simulink model "FinalDJ"  (R2017a)
settings: Solver=VariableStepAuto  StartTime=0.0  StopTime=1000  RelTol=1e-3
undefined symbols (not defined in the file): fdesignblkfcn, gcbh
libraries: dspvision x4, dspsrcs4 x3, dspsigops x3, dspobslib x2
settings Model: Creator=ilyas  LastModifiedBy=ilyas

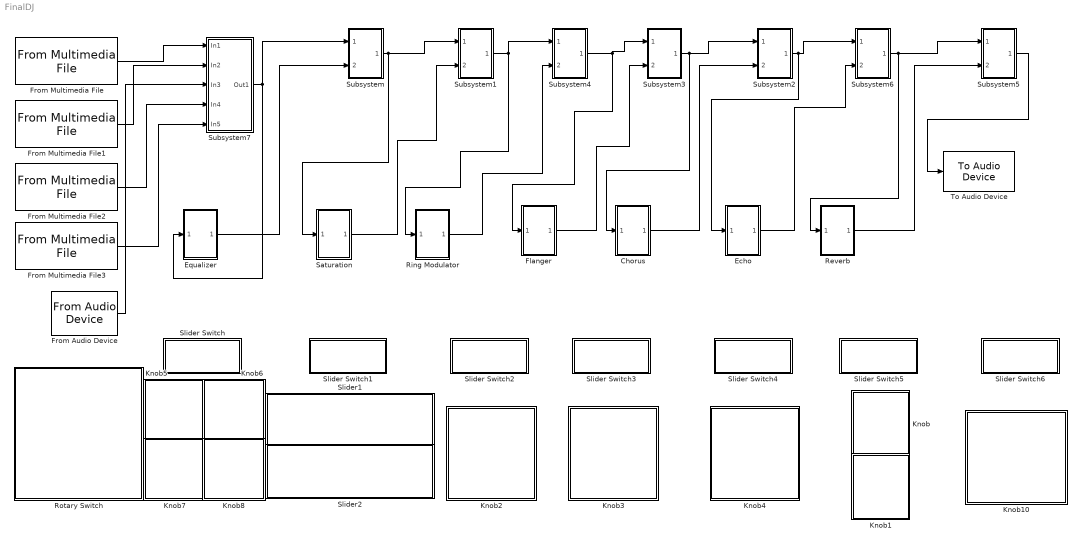
== system FinalDJ ==
  Chorus : Subsystem
  Echo : Subsystem
  Equalizer : Subsystem
  "Flanger " : Subsystem
  From Audio Device : dspobslib/From Audio Device  deviceName=Default  numChannels=1  sampleRate=44100  deviceDatatype=Determine from output data type  autoBufferSize=on  bufferSize=4096  queueDuration=1.0  frameSize=1024  outputDatatype=double  defaultInputChannelMapping=on  inputChannelMapping=1:2  outputNumOverrunSamples=off  OutputFrames=on
      settings: SourceProductName=DSP System Toolbox  SourceProductBaseCode=DS
  From Multimedia File : dspvision/From Multimedia File  inputFilename=C:\Users\ilyas\Desktop\cours UPMC\Son et image\audio\tpaudio\Tennessee-Whiskey-Cover-Instrumental-In-the-Style-.wav  loop=on  numPlays=inf  outputStreams=Audio only  videoDataType=single  audioDataType=double  inheritSampleTime=on  userDefinedSampleTime=1/30  noAudioOutput=off  isIntensityVideo=off  fourcc=RGB  colorVideoFormat=Separate color signals  outputEOF=off  dataOrg=Column-major  audioFrameSize=1024  computeAudioFrameSize=off  outSamplingMode=Sample based
      settings: SourceProductBaseCode=VP
  From Multimedia File1 : dspvision/From Multimedia File  inputFilename=C:\Users\ilyas\Desktop\cours UPMC\Son et image\audio\tpaudio\Comfortably_Numb_Pink_Floyd_Instrumental_Version_H.wav  loop=on  numPlays=inf  outputStreams=Audio only  videoDataType=single  audioDataType=double  inheritSampleTime=on  userDefinedSampleTime=1/30  noAudioOutput=off  isIntensityVideo=off  fourcc=RGB  colorVideoFormat=Separate color signals  outputEOF=off  dataOrg=Column-major  audioFrameSize=1024  computeAudioFrameSize=off  outSamplingMode=Sample based
      settings: SourceProductBaseCode=VP
  From Multimedia File2 : dspvision/From Multimedia File  inputFilename=C:\Users\ilyas\Desktop\cours UPMC\Son et image\audio\tpaudio\Perfect-Higher-Key-of-C-Piano-Karaoke-Instrumental.wav  loop=on  numPlays=inf  outputStreams=Audio only  videoDataType=single  audioDataType=double  inheritSampleTime=on  userDefinedSampleTime=1/30  noAudioOutput=off  isIntensityVideo=off  fourcc=RGB  colorVideoFormat=Separate color signals  outputEOF=off  dataOrg=Column-major  audioFrameSize=1024  computeAudioFrameSize=off  outSamplingMode=Sample based
      settings: SourceProductBaseCode=VP
  From Multimedia File3 : dspvision/From Multimedia File  inputFilename=C:\Users\ilyas\Desktop\cours UPMC\Son et image\audio\tpaudio\guitare.wav  loop=on  numPlays=inf  outputStreams=Audio only  videoDataType=single  audioDataType=double  inheritSampleTime=on  userDefinedSampleTime=1/30  noAudioOutput=off  isIntensityVideo=off  fourcc=RGB  colorVideoFormat=Separate color signals  outputEOF=off  dataOrg=Column-major  audioFrameSize=1024  computeAudioFrameSize=off  outSamplingMode=Sample based
      settings: SourceProductBaseCode=VP
  Knob : Subsystem  DialogController=hmiCreateDDGDialog  IsWebBlock=on  mask(MWDashboardBlock){webBlockId=d630c6b4-3853-4240-8efb-5ef3cca1801c, webBlockType=continuousknob, ShowInLibBrowser=on, ShowInitialText=on, HMISrcModelName=FinalDJ}
      mask prompts: webBlockId "WebBlock Id"; webBlockType "WebBlock Type"; HMISrcModelName "Source Model"
      mask help: SimulinkHMI:dialogs:ContinuousKnobDialogDesc
      mask Help: helpview([docroot '/mapfiles/simulink.map'], 'hmi_knob')
      mask Display:
      | if strcmp(get_param(bdroot(gcb),'BlockDiagramType'), 'library')
      |     image([(matlabroot) '/toolbox/simulink/hmi/icons/ContinuousKnob.png']);
      | end
  Knob1 : Subsystem  DialogController=hmiCreateDDGDialog  IsWebBlock=on  mask(MWDashboardBlock){webBlockId=0aec4347-f074-4d74-93b3-8d8c0f22ff46, webBlockType=continuousknob, ShowInLibBrowser=on, ShowInitialText=on, HMISrcModelName=FinalDJ}
      mask prompts: webBlockId "WebBlock Id"; webBlockType "WebBlock Type"; HMISrcModelName "Source Model"
      mask help: SimulinkHMI:dialogs:ContinuousKnobDialogDesc
      mask Help: helpview([docroot '/mapfiles/simulink.map'], 'hmi_knob')
      mask Display:
      | if strcmp(get_param(bdroot(gcb),'BlockDiagramType'), 'library')
      |     image([(matlabroot) '/toolbox/simulink/hmi/icons/ContinuousKnob.png']);
      | end
  Knob10 : Subsystem  DialogController=hmiCreateDDGDialog  IsWebBlock=on  mask(MWDashboardBlock){webBlockId=4e79f102-dad1-4d7d-9218-5af4294fe18a, webBlockType=continuousknob, ShowInLibBrowser=on, ShowInitialText=on, HMISrcModelName=FinalDJ}
      mask prompts: webBlockId "WebBlock Id"; webBlockType "WebBlock Type"; HMISrcModelName "Source Model"
      mask Help: helpview([docroot '/mapfiles/simulink.map'], 'hmi_knob')
      mask Display:
      | if strcmp(get_param(bdroot(gcb),'BlockDiagramType'), 'library')
      |     image([(matlabroot) '/toolbox/simulink/hmi/icons/ContinuousKnob.png']);
      | end
  Knob2 : Subsystem  DialogController=hmiCreateDDGDialog  IsWebBlock=on  mask(MWDashboardBlock){webBlockId=7d11c1b0-9d79-421c-bd63-6e862e6bd707, webBlockType=continuousknob, ShowInLibBrowser=on, ShowInitialText=on, HMISrcModelName=FinalDJ}
      mask prompts: webBlockId "WebBlock Id"; webBlockType "WebBlock Type"; HMISrcModelName "Source Model"
      mask help: SimulinkHMI:dialogs:ContinuousKnobDialogDesc
      mask Help: helpview([docroot '/mapfiles/simulink.map'], 'hmi_knob')
      mask Display:
      | if strcmp(get_param(bdroot(gcb),'BlockDiagramType'), 'library')
      |     image([(matlabroot) '/toolbox/simulink/hmi/icons/ContinuousKnob.png']);
      | end
  Knob3 : Subsystem  DialogController=hmiCreateDDGDialog  IsWebBlock=on  mask(MWDashboardBlock){webBlockId=41dfc1c3-3217-4a37-bd27-ffe62e9a6d62, webBlockType=continuousknob, ShowInLibBrowser=on, ShowInitialText=on, HMISrcModelName=FinalDJ}
      mask prompts: webBlockId "WebBlock Id"; webBlockType "WebBlock Type"; HMISrcModelName "Source Model"
      mask help: SimulinkHMI:dialogs:ContinuousKnobDialogDesc
      mask Help: helpview([docroot '/mapfiles/simulink.map'], 'hmi_knob')
      mask Display:
      | if strcmp(get_param(bdroot(gcb),'BlockDiagramType'), 'library')
      |     image([(matlabroot) '/toolbox/simulink/hmi/icons/ContinuousKnob.png']);
      | end
  Knob4 : Subsystem  DialogController=hmiCreateDDGDialog  IsWebBlock=on  mask(MWDashboardBlock){webBlockId=8e0c0283-e84a-4299-8100-d9998a7fb2dd, webBlockType=continuousknob, ShowInLibBrowser=on, ShowInitialText=on, HMISrcModelName=FinalDJ}
      mask prompts: webBlockId "WebBlock Id"; webBlockType "WebBlock Type"; HMISrcModelName "Source Model"
      mask help: SimulinkHMI:dialogs:ContinuousKnobDialogDesc
      mask Help: helpview([docroot '/mapfiles/simulink.map'], 'hmi_knob')
      mask Display:
      | if strcmp(get_param(bdroot(gcb),'BlockDiagramType'), 'library')
      |     image([(matlabroot) '/toolbox/simulink/hmi/icons/ContinuousKnob.png']);
      | end
  Knob5 : Subsystem  DialogController=hmiCreateDDGDialog  IsWebBlock=on  mask(MWDashboardBlock){webBlockId=94b2984c-17f4-476f-b59b-176a35d0d3c5, webBlockType=continuousknob, ShowInLibBrowser=on, ShowInitialText=on, HMISrcModelName=FinalDJ}
      mask prompts: webBlockId "WebBlock Id"; webBlockType "WebBlock Type"; HMISrcModelName "Source Model"
      mask Help: helpview([docroot '/mapfiles/simulink.map'], 'hmi_knob')
      mask Display:
      | if strcmp(get_param(bdroot(gcb),'BlockDiagramType'), 'library')
      |     image([(matlabroot) '/toolbox/simulink/hmi/icons/ContinuousKnob.png']);
      | end
  Knob6 : Subsystem  DialogController=hmiCreateDDGDialog  IsWebBlock=on  mask(MWDashboardBlock){webBlockId=d0e59a15-6acd-4f4b-81b9-54c366644b05, webBlockType=continuousknob, ShowInLibBrowser=on, ShowInitialText=on, HMISrcModelName=FinalDJ}
      mask prompts: webBlockId "WebBlock Id"; webBlockType "WebBlock Type"; HMISrcModelName "Source Model"
      mask Help: helpview([docroot '/mapfiles/simulink.map'], 'hmi_knob')
      mask Display:
      | if strcmp(get_param(bdroot(gcb),'BlockDiagramType'), 'library')
      |     image([(matlabroot) '/toolbox/simulink/hmi/icons/ContinuousKnob.png']);
      | end
  Knob7 : Subsystem  DialogController=hmiCreateDDGDialog  IsWebBlock=on  mask(MWDashboardBlock){webBlockId=b6ceef32-bd54-4c2a-823b-604c70b4c132, webBlockType=continuousknob, ShowInLibBrowser=on, ShowInitialText=on, HMISrcModelName=FinalDJ}
      mask prompts: webBlockId "WebBlock Id"; webBlockType "WebBlock Type"; HMISrcModelName "Source Model"
      mask Help: helpview([docroot '/mapfiles/simulink.map'], 'hmi_knob')
      mask Display:
      | if strcmp(get_param(bdroot(gcb),'BlockDiagramType'), 'library')
      |     image([(matlabroot) '/toolbox/simulink/hmi/icons/ContinuousKnob.png']);
      | end
  Knob8 : Subsystem  DialogController=hmiCreateDDGDialog  IsWebBlock=on  mask(MWDashboardBlock){webBlockId=3172c93d-703c-4a19-8532-06843a97dd04, webBlockType=continuousknob, ShowInLibBrowser=on, ShowInitialText=on, HMISrcModelName=FinalDJ}
      mask prompts: webBlockId "WebBlock Id"; webBlockType "WebBlock Type"; HMISrcModelName "Source Model"
      mask Help: helpview([docroot '/mapfiles/simulink.map'], 'hmi_knob')
      mask Display:
      | if strcmp(get_param(bdroot(gcb),'BlockDiagramType'), 'library')
      |     image([(matlabroot) '/toolbox/simulink/hmi/icons/ContinuousKnob.png']);
      | end
  Reverb : Subsystem
  Ring Modulator : Subsystem
  Rotary Switch : Subsystem  DialogController=hmiCreateDDGDialog  IsWebBlock=on  mask(MWDashboardBlock){webBlockId=78dc4692-3146-400f-aaea-232bc4b87b2b, webBlockType=discreteknob, ShowInLibBrowser=on, ShowInitialText=on, HMISrcModelName=FinalDJ}
      mask prompts: webBlockId "WebBlock Id"; webBlockType "WebBlock Type"; HMISrcModelName "Source Model"
      mask help: SimulinkHMI:dialogs:DiscreteKnobDialogDesc
      mask Help: helpview([docroot '/mapfiles/simulink.map'], 'hmi_rotary_switch')
      mask Display:
      | model = bdroot(gcb);
      | if strcmp(get_param(model,'BlockDiagramType'), 'library')
      |     image([(matlabroot) '/toolbox/simulink/hmi/icons/DiscreteKnob.png']);
      | end
  Saturation : Subsystem
  Slider Switch : Subsystem  DialogController=hmiCreateDDGDialog  IsWebBlock=on  mask(MWDashboardBlock){webBlockId=4ada6905-96e7-4612-8bb3-0a63882c9b50, webBlockType=sliderswitch, ShowInLibBrowser=on, ShowInitialText=on, HMISrcModelName=FinalDJ}
      mask prompts: webBlockId "WebBlock Id"; webBlockType "WebBlock Type"; HMISrcModelName "Source Model"
      mask help: SimulinkHMI:dialogs:SwitchDialogDesc
      mask Help: helpview([docroot '/mapfiles/simulink.map'], 'hmi_slider_switch')
      mask Display:
      | if strcmp(get_param(bdroot(gcb),'BlockDiagramType'), 'library')
      |     image([(matlabroot) '/toolbox/simulink/hmi/icons/SliderSwitch.png']);
      | end
  Slider Switch1 : Subsystem  DialogController=hmiCreateDDGDialog  IsWebBlock=on  mask(MWDashboardBlock){webBlockId=a01e8a42-961a-4294-8ccc-578b2a323852, webBlockType=sliderswitch, ShowInLibBrowser=on, ShowInitialText=on, HMISrcModelName=FinalDJ}
      mask prompts: webBlockId "WebBlock Id"; webBlockType "WebBlock Type"; HMISrcModelName "Source Model"
      mask help: SimulinkHMI:dialogs:SwitchDialogDesc
      mask Help: helpview([docroot '/mapfiles/simulink.map'], 'hmi_slider_switch')
      mask Display:
      | if strcmp(get_param(bdroot(gcb),'BlockDiagramType'), 'library')
      |     image([(matlabroot) '/toolbox/simulink/hmi/icons/SliderSwitch.png']);
      | end
  Slider Switch2 : Subsystem  DialogController=hmiCreateDDGDialog  IsWebBlock=on  mask(MWDashboardBlock){webBlockId=5848b43d-786a-4fc6-8b86-3c894cb08726, webBlockType=sliderswitch, ShowInLibBrowser=on, ShowInitialText=on, HMISrcModelName=FinalDJ}
      mask prompts: webBlockId "WebBlock Id"; webBlockType "WebBlock Type"; HMISrcModelName "Source Model"
      mask help: SimulinkHMI:dialogs:SwitchDialogDesc
      mask Help: helpview([docroot '/mapfiles/simulink.map'], 'hmi_slider_switch')
      mask Display:
      | if strcmp(get_param(bdroot(gcb),'BlockDiagramType'), 'library')
      |     image([(matlabroot) '/toolbox/simulink/hmi/icons/SliderSwitch.png']);
      | end
  Slider Switch3 : Subsystem  DialogController=hmiCreateDDGDialog  IsWebBlock=on  mask(MWDashboardBlock){webBlockId=613e13be-6908-40c7-a340-3e162b5e60f6, webBlockType=sliderswitch, ShowInLibBrowser=on, ShowInitialText=on, HMISrcModelName=FinalDJ}
      mask prompts: webBlockId "WebBlock Id"; webBlockType "WebBlock Type"; HMISrcModelName "Source Model"
      mask help: SimulinkHMI:dialogs:SwitchDialogDesc
      mask Help: helpview([docroot '/mapfiles/simulink.map'], 'hmi_slider_switch')
      mask Display:
      | if strcmp(get_param(bdroot(gcb),'BlockDiagramType'), 'library')
      |     image([(matlabroot) '/toolbox/simulink/hmi/icons/SliderSwitch.png']);
      | end
  Slider Switch4 : Subsystem  DialogController=hmiCreateDDGDialog  IsWebBlock=on  mask(MWDashboardBlock){webBlockId=eefc75fa-b4af-4e12-8e7d-34e2f9e4091e, webBlockType=sliderswitch, ShowInLibBrowser=on, ShowInitialText=on, HMISrcModelName=FinalDJ}
      mask prompts: webBlockId "WebBlock Id"; webBlockType "WebBlock Type"; HMISrcModelName "Source Model"
      mask help: SimulinkHMI:dialogs:SwitchDialogDesc
      mask Help: helpview([docroot '/mapfiles/simulink.map'], 'hmi_slider_switch')
      mask Display:
      | if strcmp(get_param(bdroot(gcb),'BlockDiagramType'), 'library')
      |     image([(matlabroot) '/toolbox/simulink/hmi/icons/SliderSwitch.png']);
      | end
  Slider Switch5 : Subsystem  DialogController=hmiCreateDDGDialog  IsWebBlock=on  mask(MWDashboardBlock){webBlockId=c9b1026d-64ff-488d-90fa-6a40fe1ec0ef, webBlockType=sliderswitch, ShowInLibBrowser=on, ShowInitialText=on, HMISrcModelName=FinalDJ}
      mask prompts: webBlockId "WebBlock Id"; webBlockType "WebBlock Type"; HMISrcModelName "Source Model"
      mask help: SimulinkHMI:dialogs:SwitchDialogDesc
      mask Help: helpview([docroot '/mapfiles/simulink.map'], 'hmi_slider_switch')
      mask Display:
      | if strcmp(get_param(bdroot(gcb),'BlockDiagramType'), 'library')
      |     image([(matlabroot) '/toolbox/simulink/hmi/icons/SliderSwitch.png']);
      | end
  Slider Switch6 : Subsystem  DialogController=hmiCreateDDGDialog  IsWebBlock=on  mask(MWDashboardBlock){webBlockId=73165ce2-164f-4206-9756-31df083dc0b7, webBlockType=sliderswitch, ShowInLibBrowser=on, ShowInitialText=on, HMISrcModelName=FinalDJ}
      mask prompts: webBlockId "WebBlock Id"; webBlockType "WebBlock Type"; HMISrcModelName "Source Model"
      mask help: SimulinkHMI:dialogs:SwitchDialogDesc
      mask Help: helpview([docroot '/mapfiles/simulink.map'], 'hmi_slider_switch')
      mask Display:
      | if strcmp(get_param(bdroot(gcb),'BlockDiagramType'), 'library')
      |     image([(matlabroot) '/toolbox/simulink/hmi/icons/SliderSwitch.png']);
      | end
  Slider1 : Subsystem  DialogController=hmiCreateDDGDialog  IsWebBlock=on  mask(MWDashboardBlock){webBlockId=dbaf6efe-b768-4b21-a436-d0de633b73bf, webBlockType=slider, ShowInLibBrowser=on, ShowInitialText=on, HMISrcModelName=FinalDJ}
      mask prompts: webBlockId "WebBlock Id"; webBlockType "WebBlock Type"; HMISrcModelName "Source Model"
      mask help: SimulinkHMI:dialogs:SliderDialogDesc
      mask Help: helpview([docroot '/mapfiles/simulink.map'], 'hmi_slider')
      mask Display:
      | if strcmp(get_param(bdroot(gcb),'BlockDiagramType'), 'library')
      |     image([(matlabroot) '/toolbox/simulink/hmi/icons/Slider.png']);
      | end
  Slider2 : Subsystem  DialogController=hmiCreateDDGDialog  IsWebBlock=on  mask(MWDashboardBlock){webBlockId=232908e4-0a8b-4e56-856e-cf1bb558e568, webBlockType=slider, ShowInLibBrowser=on, ShowInitialText=on, HMISrcModelName=FinalDJ}
      mask prompts: webBlockId "WebBlock Id"; webBlockType "WebBlock Type"; HMISrcModelName "Source Model"
      mask help: SimulinkHMI:dialogs:SliderDialogDesc
      mask Help: helpview([docroot '/mapfiles/simulink.map'], 'hmi_slider')
      mask Display:
      | if strcmp(get_param(bdroot(gcb),'BlockDiagramType'), 'library')
      |     image([(matlabroot) '/toolbox/simulink/hmi/icons/Slider.png']);
      | end
  Subsystem : Subsystem
  Subsystem1 : Subsystem
  Subsystem2 : Subsystem
  Subsystem3 : Subsystem
  Subsystem4 : Subsystem
  Subsystem5 : Subsystem
  Subsystem6 : Subsystem
  Subsystem7 : Subsystem
  To Audio Device : dspobslib/To Audio Device  deviceName=Default  inheritSampleRate=on  sampleRate=11025  deviceDatatype=Determine from input data type  autoBufferSize=on  bufferSize=2048  queueDuration=1.0  defaultOutputChannelMapping=on  outputChannelMapping=1:2  outputNumUnderrunSamples=off
      settings: SourceProductName=DSP System Toolbox  SourceProductBaseCode=DS
  wires:
  Subsystem1/1(Out1) -> Subsystem4/1(In1), Ring Modulator/1(In1)
  Subsystem4/1(Out1) -> Subsystem3/1(In1), "Flanger "/1(In1)
  Subsystem3/1(Out1) -> Chorus/1(In1), Subsystem2/1(In1)
  Subsystem2/1(Out1) -> Subsystem6/1(In1), Echo/1(In1)
  Subsystem6/1(Out1) -> Subsystem5/1(In1), Reverb/1(In1)
  Reverb/1(Out1) -> Subsystem5/2(In2)
  Subsystem/1(Out1) -> Subsystem1/1(In1), Saturation/1(In1)
  Equalizer/1(Out1) -> Subsystem/2(In2)
  Saturation/1(Out1) -> Subsystem1/2(In2)
  Ring Modulator/1(Out1) -> Subsystem4/2(In2)
  "Flanger "/1(Out1) -> Subsystem3/2(In2)
  Chorus/1(Out1) -> Subsystem2/2(In2)
  Echo/1(Out1) -> Subsystem6/2(In2)
  Subsystem5/1(Out1) -> To Audio Device/1
  Subsystem7/1(Out1) -> Subsystem/1(In1), Equalizer/1(In1)
  From Multimedia File/1 -> Subsystem7/1(In1)
  From Multimedia File1/1 -> Subsystem7/2(In2)
  From Multimedia File2/1 -> Subsystem7/4(In4)
  From Multimedia File3/1 -> Subsystem7/5(In5)
  From Audio Device/1 -> Subsystem7/3(In3)

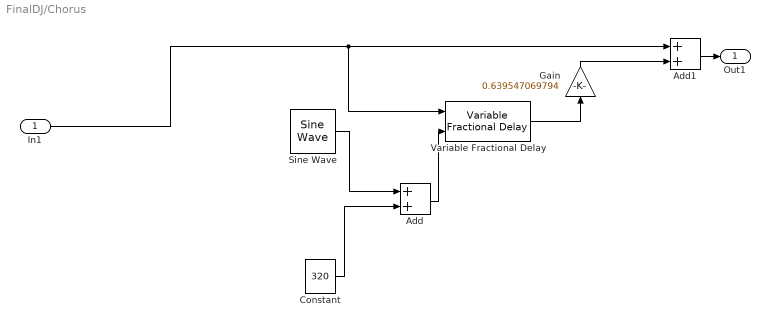
== system FinalDJ/Chorus ==
  In1 : Inport
  Add : Sum
  Add1 : Sum
  Constant : Constant  Value=320  VectorParams1D=off
  Gain : Gain  Gain=0.639547069794
  Sine Wave : dspsrcs4/Sine Wave  Amplitude=80  Frequency=0.7  Phase=0  SampleMode=Discrete  OutComplex=Real  CompMethod=Trigonometric fcn  TableSize=Speed  SampleTime=1/44100  SamplesPerFrame=1024  ResetState=Restart at time zero  OutputFrames=off  dataType=double  wordLen=16  udDataType=sfix(16)  fracBitsMode=Best precision  numFracBits=15  OutDataTypeStr=double  LastOutDataTypeStr=double
  Variable Fractional Delay : dspsigops/Variable Fractional Delay  mode=OBSOLETE  modeActive=Linear  dmax=10000  InputProcessing=Columns as channels (frame based)  L=4  FarrowL=4  R=10  alpha=1  ic=0  fallbackFIR=Clip to the minimum value necessary for centered kernel  fallbackFarrow=Clip to the minimum value necessary for centered kernel  noDFT=off  roundingMode=Zero  overflowMode=off
      settings: SourceProductName=DSP System Toolbox  SourceProductBaseCode=DS
  Out1 : Outport
  wires:
  Gain/1 -> Add1/2
  In1/1 -> Add1/1, Variable Fractional Delay/1
  Constant/1 -> Add/2
  Variable Fractional Delay/1 -> Gain/1
  Sine Wave/1 -> Add/1
  Add/1 -> Variable Fractional Delay/2
  Add1/1 -> Out1/1

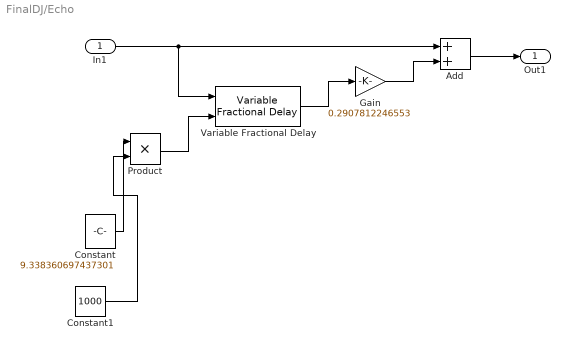
== system FinalDJ/Echo ==
  In1 : Inport
  Add : Sum
  Constant : Constant  Value=9.338360697437301  VectorParams1D=off
  Constant1 : Constant  Value=1000
  Gain : Gain  Gain=0.2907812246553
  Product : Product
  Variable Fractional Delay : dspsigops/Variable Fractional Delay  mode=OBSOLETE  modeActive=Linear  dmax=11000  InputProcessing=Columns as channels (frame based)  L=4  FarrowL=4  R=10  alpha=1  ic=0  fallbackFIR=Clip to the minimum value necessary for centered kernel  fallbackFarrow=Clip to the minimum value necessary for centered kernel  noDFT=off  roundingMode=Zero  overflowMode=off
      settings: SourceProductName=DSP System Toolbox  SourceProductBaseCode=DS
  Out1 : Outport
  wires:
  Gain/1 -> Add/2
  In1/1 -> Variable Fractional Delay/1, Add/1
  Variable Fractional Delay/1 -> Gain/1
  Add/1 -> Out1/1
  Constant/1 -> Product/1
  Constant1/1 -> Product/2
  Product/1 -> Variable Fractional Delay/2

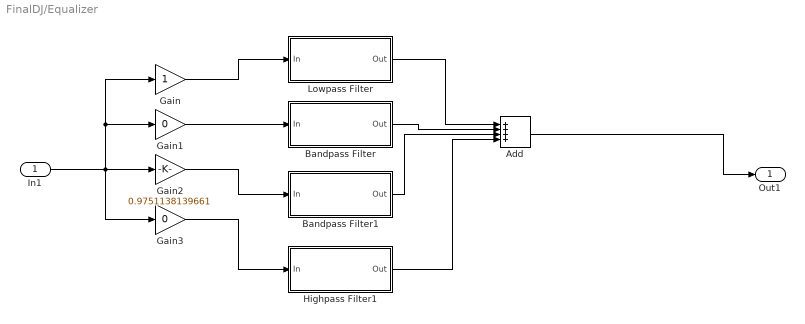
== system FinalDJ/Equalizer ==
  In1 : Inport
  Add : Sum  Inputs=++++
  Bandpass Filter : Subsystem  DialogController=fdesignblkfcn  InitFcn=fdesignblkfcn(gcbh, {'InitFcn'});  mask(Bandpass Filter){}
      mask help: Design a bandpass filter
      settings: CopyFcn=fdesignblkfcn(gcbh, {'CopyFcn'});
      mask Help: helpview(mapfilelocation('dsp'), 'dspbandpassfilter');
      mask Display: disp('Bandpass');
  Bandpass Filter1 : Subsystem  DialogController=fdesignblkfcn  InitFcn=fdesignblkfcn(gcbh, {'InitFcn'});  mask(Bandpass Filter){}
      mask help: Design a bandpass filter
      settings: CopyFcn=fdesignblkfcn(gcbh, {'CopyFcn'});
      mask Help: helpview(mapfilelocation('dsp'), 'dspbandpassfilter');
      mask Display: disp('Bandpass');
  Gain : Gain
  Gain1 : Gain  Gain=0
  Gain2 : Gain  Gain=0.9751138139661
  Gain3 : Gain  Gain=0
  Highpass Filter1 : Subsystem  DialogController=fdesignblkfcn  InitFcn=fdesignblkfcn(gcbh, {'InitFcn'});  mask(Highpass Filter){}
      mask help: Design a highpass filter
      settings: CopyFcn=fdesignblkfcn(gcbh, {'CopyFcn'});
      mask Help: helpview(mapfilelocation('dsp'), 'dsphighpassfilter');
      mask Display: disp('Highpass')
  Lowpass Filter : Subsystem  DialogController=fdesignblkfcn  InitFcn=fdesignblkfcn(gcbh, {'InitFcn'});  mask(Lowpass Filter){}
      mask help: Design a lowpass filter
      settings: CopyFcn=fdesignblkfcn(gcbh, {'CopyFcn'});
      mask Help: helpview(mapfilelocation('dsp'), 'dsplowpassfilter');
      mask Display: disp('Lowpass')
  Out1 : Outport
  wires:
  In1/1 -> Gain3/1, Gain1/1, Gain/1, Gain2/1
  Gain/1 -> Lowpass Filter/1(In)
  Gain1/1 -> Bandpass Filter/1(In)
  Gain2/1 -> Bandpass Filter1/1(In)
  Gain3/1 -> Highpass Filter1/1(In)
  Lowpass Filter/1(Out) -> Add/1
  Bandpass Filter/1(Out) -> Add/2
  Bandpass Filter1/1(Out) -> Add/3
  Highpass Filter1/1(Out) -> Add/4
  Add/1 -> Out1/1

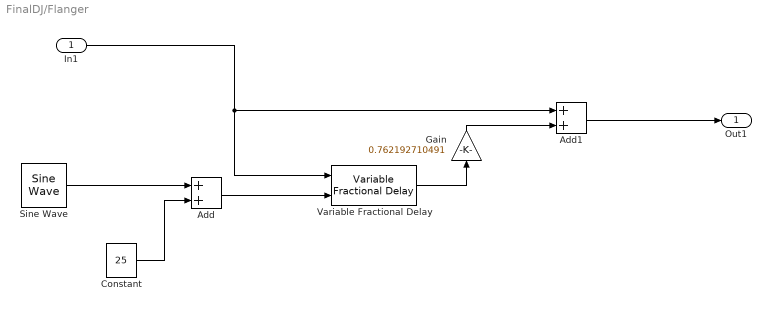
== system FinalDJ/Flanger  ==
  In1 : Inport
  Add : Sum
  Add1 : Sum
  Constant : Constant  Value=25  VectorParams1D=off
  Gain : Gain  Gain=0.762192710491
  Sine Wave : dspsrcs4/Sine Wave  Amplitude=20  Frequency=0.7  Phase=0  SampleMode=Discrete  OutComplex=Real  CompMethod=Trigonometric fcn  TableSize=Speed  SampleTime=1/44100  SamplesPerFrame=1024  ResetState=Restart at time zero  OutputFrames=off  dataType=double  wordLen=16  udDataType=sfix(16)  fracBitsMode=Best precision  numFracBits=15  OutDataTypeStr=double  LastOutDataTypeStr=double
  Variable Fractional Delay : dspsigops/Variable Fractional Delay  mode=OBSOLETE  modeActive=Linear  dmax=10000  InputProcessing=Columns as channels (frame based)  L=4  FarrowL=4  R=10  alpha=1  ic=0  fallbackFIR=Clip to the minimum value necessary for centered kernel  fallbackFarrow=Clip to the minimum value necessary for centered kernel  noDFT=off  roundingMode=Zero  overflowMode=off
      settings: SourceProductName=DSP System Toolbox  SourceProductBaseCode=DS
  Out1 : Outport
  wires:
  Sine Wave/1 -> Add/1
  Add/1 -> Variable Fractional Delay/2
  Constant/1 -> Add/2
  In1/1 -> Add1/1, Variable Fractional Delay/1
  Variable Fractional Delay/1 -> Gain/1
  Add1/1 -> Out1/1
  Gain/1 -> Add1/2

== system FinalDJ/Knob ==

== system FinalDJ/Knob1 ==

== system FinalDJ/Knob10 ==

== system FinalDJ/Knob2 ==

== system FinalDJ/Knob3 ==

== system FinalDJ/Knob4 ==

== system FinalDJ/Knob5 ==

== system FinalDJ/Knob6 ==

== system FinalDJ/Knob7 ==

== system FinalDJ/Knob8 ==

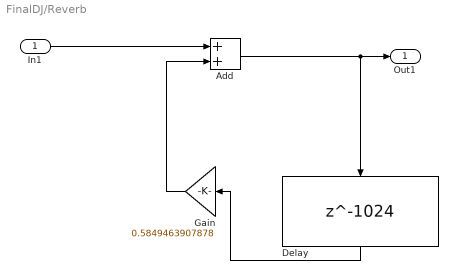
== system FinalDJ/Reverb ==
  In1 : Inport
  Add : Sum
  Delay : Delay  DelayLength=1024  DelayLengthUpperLimit=5000  InitialCondition=4000  InputProcessing=Columns as channels (frame based)
  Gain : Gain  Gain=0.5849463907878
  Out1 : Outport
  wires:
  Gain/1 -> Add/2
  Add/1 -> Out1/1, Delay/1
  Delay/1 -> Gain/1
  In1/1 -> Add/1

== system FinalDJ/Ring Modulator ==
  In1 : Inport
  Product : Product
  Sine Wave : dspsrcs4/Sine Wave  Amplitude=1  Frequency=104.40785428156  Phase=0  SampleMode=Discrete  OutComplex=Real  CompMethod=Trigonometric fcn  TableSize=Speed  SampleTime=1/44100  SamplesPerFrame=1024  ResetState=Restart at time zero  OutputFrames=off  dataType=double  wordLen=16  udDataType=sfix(16)  fracBitsMode=Best precision  numFracBits=15  OutDataTypeStr=double  LastOutDataTypeStr=double
  Out1 : Outport
  wires:
  Sine Wave/1 -> Product/2
  In1/1 -> Product/1
  Product/1 -> Out1/1

== system FinalDJ/Rotary Switch ==

== system FinalDJ/Saturation ==
  In1 : Inport
  Saturation : Saturate  UpperLimit=1.9121301775148  LowerLimit=-2.100591715976
  Out1 : Outport
  wires:
  Saturation/1 -> Out1/1
  In1/1 -> Saturation/1

== system FinalDJ/Slider Switch ==

== system FinalDJ/Slider Switch1 ==

== system FinalDJ/Slider Switch2 ==

== system FinalDJ/Slider Switch3 ==

== system FinalDJ/Slider Switch4 ==

== system FinalDJ/Slider Switch5 ==

== system FinalDJ/Slider Switch6 ==

== system FinalDJ/Slider1 ==

== system FinalDJ/Slider2 ==

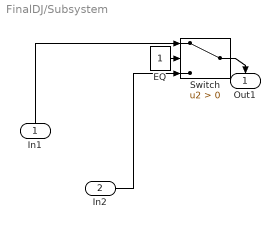
== system FinalDJ/Subsystem ==
  In1 : Inport
  In2 : Inport  Port=2
  EQ : Constant  VectorParams1D=off
  Switch : Switch  Criteria=u2 > Threshold
  Out1 : Outport
  wires:
  In2/1 -> Switch/3
  EQ/1 -> Switch/2
  In1/1 -> Switch/1
  Switch/1 -> Out1/1

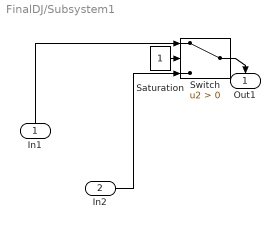
== system FinalDJ/Subsystem1 ==
  In1 : Inport
  In2 : Inport  Port=2
  Saturation : Constant  VectorParams1D=off
  Switch : Switch  Criteria=u2 > Threshold
  Out1 : Outport
  wires:
  Switch/1 -> Out1/1
  In1/1 -> Switch/1
  Saturation/1 -> Switch/2
  In2/1 -> Switch/3

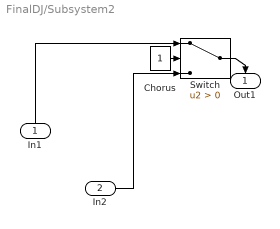
== system FinalDJ/Subsystem2 ==
  In1 : Inport
  In2 : Inport  Port=2
  Chorus : Constant  VectorParams1D=off
  Switch : Switch  Criteria=u2 > Threshold
  Out1 : Outport
  wires:
  In2/1 -> Switch/3
  Chorus/1 -> Switch/2
  In1/1 -> Switch/1
  Switch/1 -> Out1/1

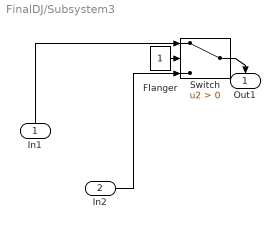
== system FinalDJ/Subsystem3 ==
  In1 : Inport
  In2 : Inport  Port=2
  Flanger : Constant  VectorParams1D=off
  Switch : Switch  Criteria=u2 > Threshold
  Out1 : Outport
  wires:
  Switch/1 -> Out1/1
  In1/1 -> Switch/1
  Flanger/1 -> Switch/2
  In2/1 -> Switch/3

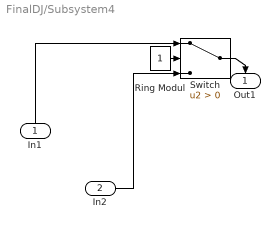
== system FinalDJ/Subsystem4 ==
  In1 : Inport
  In2 : Inport  Port=2
  Ring Modul : Constant  VectorParams1D=off
  Switch : Switch  Criteria=u2 > Threshold
  Out1 : Outport
  wires:
  In2/1 -> Switch/3
  Ring Modul/1 -> Switch/2
  In1/1 -> Switch/1
  Switch/1 -> Out1/1

== system FinalDJ/Subsystem5 ==
  In1 : Inport
  In2 : Inport  Port=2
  Reverb : Constant  VectorParams1D=off
  Switch : Switch  Criteria=u2 > Threshold
  Out1 : Outport
  wires:
  Switch/1 -> Out1/1
  In1/1 -> Switch/1
  Reverb/1 -> Switch/2
  In2/1 -> Switch/3

== system FinalDJ/Subsystem6 ==
  In1 : Inport
  In2 : Inport  Port=2
  Echo : Constant  Value=0  VectorParams1D=off
  Switch : Switch  Criteria=u2 > Threshold
  Out1 : Outport
  wires:
  In2/1 -> Switch/3
  Echo/1 -> Switch/2
  In1/1 -> Switch/1
  Switch/1 -> Out1/1

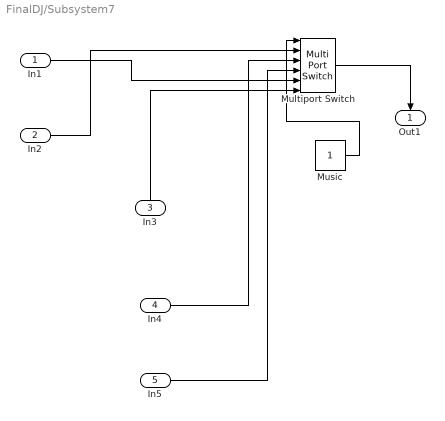
== system FinalDJ/Subsystem7 ==
  In1 : Inport
  In2 : Inport  Port=2
  In3 : Inport  Port=3
  In4 : Inport  Port=4
  In5 : Inport  Port=5
  Multiport Switch : MultiPortSwitch  Inputs=5
  Music : Constant
  Out1 : Outport
  wires:
  Music/1 -> Multiport Switch/1
  In2/1 -> Multiport Switch/2
  In1/1 -> Multiport Switch/5
  In3/1 -> Multiport Switch/6
  In5/1 -> Multiport Switch/4
  In4/1 -> Multiport Switch/3
  Multiport Switch/1 -> Out1/1

== system FinalDJ/Equalizer/Bandpass Filter ==
  In : Inport
  Generated Filter Block : DiscreteFir  Tag=BlockMethodSubSystem  Coefficients=[-0.034227365537242295 0.018312757492087928 0.05932130178861178 -0.015649458947768258 0.0096465114342621835 -0.029035785159490478 -0.015761984269044724 -0.037689628472410135 -0.03202966742034466 -0.044813544994417052 -0.042077522064569023 -0.047994018438133036 -0.044347414970127598 -0.043895492779424998 -0.036914882245408523 -0.030447360988786105 -0.019612599669352172 -0.00858331876634379 0.0047869939251154146 0.017832982590566839 0.03123510535086213 0.043139022752045862 0.053593260564708499 0.061360943995909772 0.066388263112684393 0.06800122583920179 0.066388263112684393 0.061360943995909772 0.053593260564708499 0.043139022752045862 0.03123510535086213 0.017832982590566839 0.0047869939251154146 -0.00858331876634379 -0.019612599669352172 -0.030447360988786105 -0.036914882245408523 -0.043895492779424998 -0.044347414970127598 -0.047994018438133036 -0.042077522064569023 -0.044813544994417052 -0.03202966742034466 -0.037689628472410135 -0.015761984269044724 -0.029035785159490478 0.0096465114342621835 -0.015649458947768258 0.05932130178861178 0.018312757492087928 -0.034227365537242295]  InputProcessing=Columns as channels (frame based)
  Out : Outport
  wires:
  Generated Filter Block/1 -> Out/1
  In/1 -> Generated Filter Block/1

== system FinalDJ/Equalizer/Bandpass Filter1 ==
  In : Inport
  Generated Filter Block : DiscreteFir  Tag=BlockMethodSubSystem  Coefficients=[-0.071193933975794793 0.042567551632574072 0.023370929263920877 0.0067492245502078505 -0.0056303528823154706 -0.012406515894683801 -0.012509643538729659 -0.0056607808720928483 0.0073925777727120202 0.024156862094491815 0.040950617859290002 0.05303589501571479 0.05614662588295434 0.047414277531303138 0.026950275664504888 -0.0021817284297539169 -0.033973814822860146 -0.06117405180846118 -0.076560218072753941 -0.075309696327126918 -0.056281928917521193 -0.023018521202301939 0.017523864292477515 0.056264679144848485 0.083815001474115053 0.09388074499835046 0.083815001474115053 0.056264679144848485 0.017523864292477515 -0.023018521202301939 -0.056281928917521193 -0.075309696327126918 -0.076560218072753941 -0.06117405180846118 -0.033973814822860146 -0.0021817284297539169 0.026950275664504888 0.047414277531303138 0.05614662588295434 0.05303589501571479 0.040950617859290002 0.024156862094491815 0.0073925777727120202 -0.0056607808720928483 -0.012509643538729659 -0.012406515894683801 -0.0056303528823154706 0.0067492245502078505 0.023370929263920877 0.042567551632574072 -0.071193933975794793]  InputProcessing=Columns as channels (frame based)
  Out : Outport
  wires:
  Generated Filter Block/1 -> Out/1
  In/1 -> Generated Filter Block/1

== system FinalDJ/Equalizer/Highpass Filter1 ==
  In : Inport
  Generated Filter Block : DiscreteFir  Tag=BlockMethodSubSystem  Coefficients=[0.018474008886137774 -0.07093427222798343 -0.026736009141952864 -0.012590249565781884 -0.0029223409381482746 0.0064166158658349477 0.01376997205732409 0.016707240639420411 0.013639039609664469 0.0049637238837780427 -0.0068574716590106451 -0.017827795097230564 -0.023758479772147303 -0.021504192552314477 -0.010454091224033886 0.0070581716995950124 0.025786675130562247 0.038995997151154212 0.040090951391899117 0.024873356561464898 -0.0071750444445839922 -0.052280451761689467 -0.1027024963340082 -0.14890293216856484 -0.18115471356170157 0.80737130806986068 -0.18115471356170157 -0.14890293216856484 -0.1027024963340082 -0.052280451761689467 -0.0071750444445839922 0.024873356561464898 0.040090951391899117 0.038995997151154212 0.025786675130562247 0.0070581716995950124 -0.010454091224033886 -0.021504192552314477 -0.023758479772147303 -0.017827795097230564 -0.0068574716590106451 0.0049637238837780427 0.013639039609664469 0.016707240639420411 0.01376997205732409 0.0064166158658349477 -0.0029223409381482746 -0.012590249565781884 -0.026736009141952864 -0.07093427222798343 0.018474008886137774]  InputProcessing=Columns as channels (frame based)
  Out : Outport
  wires:
  In/1 -> Generated Filter Block/1
  Generated Filter Block/1 -> Out/1

== system FinalDJ/Equalizer/Lowpass Filter ==
  In : Inport
  Generated Filter Block : DiscreteFir  Tag=BlockMethodSubSystem  Coefficients=[-0.067571599194720749 0.028366275622582534 0.024365308441611347 0.021834882196456632 0.020229321096330865 0.019593102757112429 0.019467767446300618 0.01970710174125179 0.020316328767870182 0.021189381305964993 0.022233119686554535 0.023289912862881998 0.024434404835929416 0.025590101085555161 0.026793987513412713 0.027904494200213244 0.028994063526814901 0.029963415719363243 0.030889637193174065 0.031658907557582189 0.03237246922527081 0.032938831357787801 0.033449784931778435 0.033783249602137515 0.034025406529673743 0.034071811260776463 0.034025406529673743 0.033783249602137515 0.033449784931778435 0.032938831357787801 0.03237246922527081 0.031658907557582189 0.030889637193174065 0.029963415719363243 0.028994063526814901 0.027904494200213244 0.026793987513412713 0.025590101085555161 0.024434404835929416 0.023289912862881998 0.022233119686554535 0.021189381305964993 0.020316328767870182 0.01970710174125179 0.019467767446300618 0.019593102757112429 0.020229321096330865 0.021834882196456632 0.024365308441611347 0.028366275622582534 -0.067571599194720749]  InputProcessing=Columns as channels (frame based)
  Out : Outport
  wires:
  Generated Filter Block/1 -> Out/1
  In/1 -> Generated Filter Block/1
